simulink model "untitle"  (R2019a)
settings: Solver=FixedStepAuto  StartTime=0.0  StopTime=1e4  FixedStep=0.001  RelTol=1e-3
settings Model: Creator=hebuyong  LastModifiedBy=hebuyong

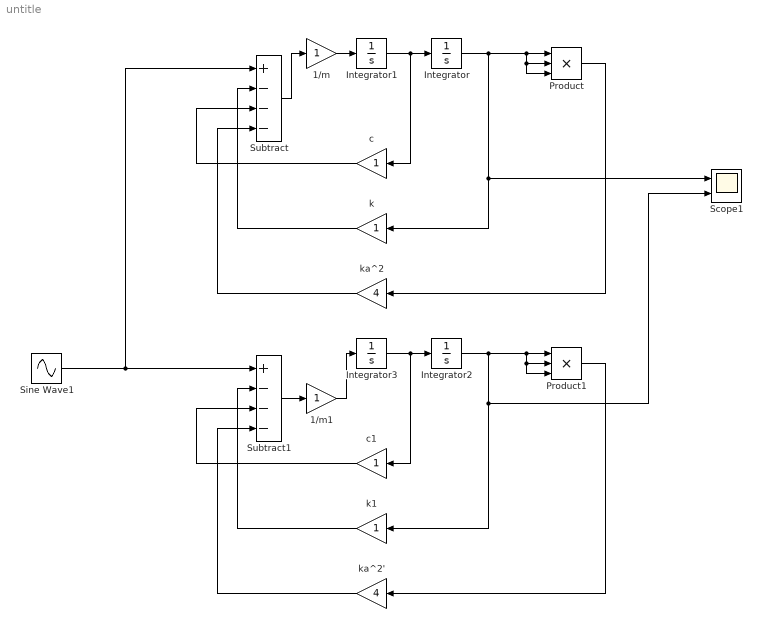
== system untitle ==
  1/m : Gain
  1/m1 : Gain
  Integrator : Integrator  InitialCondition=0.1
  Integrator1 : Integrator
  Integrator2 : Integrator  InitialCondition=0.101
  Integrator3 : Integrator
  Product : Product  Inputs=3
  Product1 : Product  Inputs=3
  Scope1 : Scope  NumInputPorts=2
  Sine Wave1 : Sin  Frequency=2*pi  Phase=-pi/2  SampleTime=0
  Subtract : Sum  Inputs=+---
  Subtract1 : Sum  Inputs=+---
  c : Gain
  c1 : Gain
  k : Gain
  k1 : Gain
  ka^2 : Gain  Gain=4
  ka^2' : Gain  Gain=4
  wires:
  Integrator/1 -> Scope1/1, k/1, Product/3, Product/2, Product/1
  Sine Wave1/1 -> Subtract/1, Subtract1/1
  k/1 -> Subtract/2
  Integrator1/1 -> c/1, Integrator/1
  c/1 -> Subtract/3
  Product/1 -> ka^2/1
  ka^2/1 -> Subtract/4
  Subtract/1 -> 1/m/1
  1/m/1 -> Integrator1/1
  1/m1/1 -> Integrator3/1
  Subtract1/1 -> 1/m1/1
  Integrator2/1 -> Scope1/2, k1/1, Product1/3, Product1/2, Product1/1
  c1/1 -> Subtract1/3
  ka^2'/1 -> Subtract1/4
  Product1/1 -> ka^2'/1
  Integrator3/1 -> c1/1, Integrator2/1
  k1/1 -> Subtract1/2
